simulink model "Ultrasonic_Ranging_Sensor0"  (R2020b)
settings: Solver=FixedStepAuto  StartTime=0.0  StopTime=2  FixedStep=1e-06  RelTol=1e-3  EnableMultiTasking=on
settings Model: SILPILModeSetting=veronly  ExtModeTrigDuration=2  Creator=GUO HUI  LastModifiedBy=GUO HUI
settings DataIOCC: SaveOutput=off  SaveTime=off
settings OptimizationCC: EnhancedBackFolding=on  PassReuseOutputArgsAs=Individual arguments  MaxStackSize=64  OptimizeBlockOrder=speed  DifferentSizesBufferReuse=on  OptimizationCustomize=off  EfficientTunableParamExpr=on
settings DebuggingCC: ParameterTunabilityLossMsg=error
settings HardwareCC: ProdBitPerInt=16  ProdBitPerPointer=16  ProdBitPerSizeT=16  ProdBitPerPtrDiffT=16  ProdLargestAtomicFloat=None  ProdWordSize=8  ProdHWDeviceType=Atmel->AVR
settings SFSimCC: MATLABDynamicMemAlloc=off
settings RTWCC: Description=Embedded Coder  SystemTargetFile=ert.tlc  HardwareBoard=Arduino Uno  TemplateMakefile=ert_default_tmf  GenerateReport=on  Toolchain=Arduino AVR  BuildConfiguration=Faster Runs  IncludeHyperlinkInReport=on  LaunchReport=on  GenerateTraceInfo=on  GenerateCodeMetricsReport=on
settings CodeAppCC: ForceParamTrailComments=on  IgnoreCustomStorageClasses=off  OperatorAnnotations=on  SimulinkDataObjDesc=on  SFDataObjDesc=on  InsertBlockDesc=on
settings ERTTargetCC: CodeInterfacePackaging=Reusable function  SupportContinuousTime=on  SupportVariableSizeSignals=on  ExtModeStaticAllocSize=250  ERTFilePackagingFormat=Compact

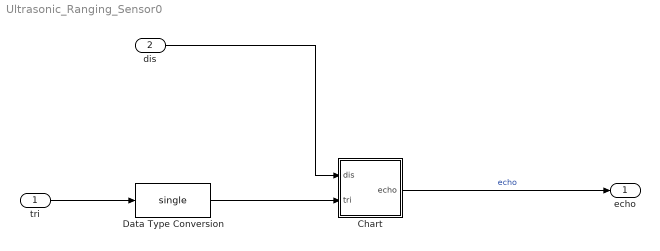
== system Ultrasonic_Ranging_Sensor0 ==
  tri : Inport  OutDataTypeStr=single  PortDimensions=1
  dis : Inport  Port=2  OutDataTypeStr=double  PortDimensions=1
  Chart : Stateflow chart  TreatAsAtomicUnit=on
  Data Type Conversion : DataTypeConversion  OutDataTypeStr=single  LockScale=on
  echo : Outport  OutDataTypeStr=double  PortDimensions=1  SampleTime=[9.9999999999999995e-07,0]
  wires:
  tri/1 -> Data Type Conversion/1
  dis/1 -> Chart/1(dis)
  Chart/1(echo) -> echo/1  "echo"
  Data Type Conversion/1 -> Chart/2(tri)

== stateflow chart Ultrasonic_Ranging_Sensor0/Chart ==
  state start
    en:echo=0
  state echo_up
    en:echo=1
    echodu=dis
  state echo_down
    en:echo=0
  echo_down -> start : [tri==0]
  (default) -> start
  echo_up -> echo_down : after(echodu*58,usec)
  start -> echo_up : [tri==1]
  data: dis input; tri input; echo output; echodu local
